simulink model "CSWI"  (Simulink 7.8)
settings: Solver=ode3  StartTime=0.0  StopTime=t_sim  FixedStep=1/6400  MaxStep=0.001  MinStep=0.000005  RelTol=1e-3
StopFcn:
  | ComtradeWrite5( RDRE1_UIabc, RDRE1_ANames, RDRE1_Dsignals, RDRE1_DNames, RDRE1_ADCscale, RDRE1_PromtFile, RDRE1_NumFile, RDRE1_FileFormat, RDRE1_TestNum);
  | clear RDRE1_UIabc RDRE1_ANames RDRE1_Dsignals RDRE1_DNames RDRE1_ADCscale  RDRE1_PromtFile RDRE1_NumFile RDRE1_FileFormat RDRE1_TestNum
values from neighbouring files (symbols this model uses):
  BlkTmms1 = 700    [CSWI_SG1.m]    (also in CSWI_SG2.m = 650; CSWI_SG3.m; CSWI_SG4.m; CSWI_SG5.m)
  BlkTmms2 = 800    [CSWI_SG1.m]    (also in CSWI_SG2.m = 750; CSWI_SG3.m; CSWI_SG4.m; CSWI_SG5.m)
  ClsTmms1 = 250    [CSWI_SG1.m]    (also in CSWI_SG2.m = 200; CSWI_SG3.m; CSWI_SG4.m; CSWI_SG5.m)
  ClsTmms2 = 170    [CSWI_SG1.m]    (also in CSWI_SG2.m = 100; CSWI_SG3.m; CSWI_SG4.m; CSWI_SG5.m)
  ClsTmms3 = 60    [CSWI_SG1.m]    (also in CSWI_SG2.m = 30; CSWI_SG3.m; CSWI_SG4.m; CSWI_SG5.m)
  ClsTmms4 = 10    [CSWI_SG1.m]    (also in CSWI_SG2.m = 20; CSWI_SG3.m; CSWI_SG4.m; CSWI_SG5.m)
  FailTmms = 350    [CSWI_SG1.m]    (also in CSWI_SG2.m = 300; CSWI_SG3.m; CSWI_SG4.m; CSWI_SG5.m)
  FctMod1 = 1    [CSWI_SG1.m]    (also in CSWI_SG2.m; CSWI_SG3.m; CSWI_SG4.m; CSWI_SG5.m)
  FctMod2 = 1    [CSWI_SG1.m]    (also in CSWI_SG2.m; CSWI_SG3.m; CSWI_SG4.m = 0; CSWI_SG5.m)
  FctMod3 = 1    [CSWI_SG1.m]    (also in CSWI_SG2.m; CSWI_SG3.m; CSWI_SG4.m; CSWI_SG5.m = 0)
  Num_SG = 1    [CSWI_generate_tests.m]
  OpnTmms1 = 300    [CSWI_SG1.m]    (also in CSWI_SG2.m = 250; CSWI_SG3.m; CSWI_SG4.m; CSWI_SG5.m)
  OpnTmms2 = 200    [CSWI_SG1.m]    (also in CSWI_SG2.m = 150; CSWI_SG3.m; CSWI_SG4.m; CSWI_SG5.m)
  OpnTmms3 = 30    [CSWI_SG1.m]    (also in CSWI_SG2.m = 90; CSWI_SG3.m = 90; CSWI_SG4.m; CSWI_SG5.m)
  test_dc = 'Ïðîâåðêà îòñóòñòâèÿ ôîðìèðîâàíèÿ ñèãíàëîâ "Âêë." ïðè ôîðìèðîâàíèè ñèãíàëà  "Îòêë. îò ÄÓ"'    [CSWI_generate_tests.m]
undefined symbols (not defined in the file or in its folder): sigbuilder_block, Test_num
libraries: powerlib_extras x21
(part 1 of 3)
settings Model: Creator=ivanovsn  LastModifiedBy=nikonenok

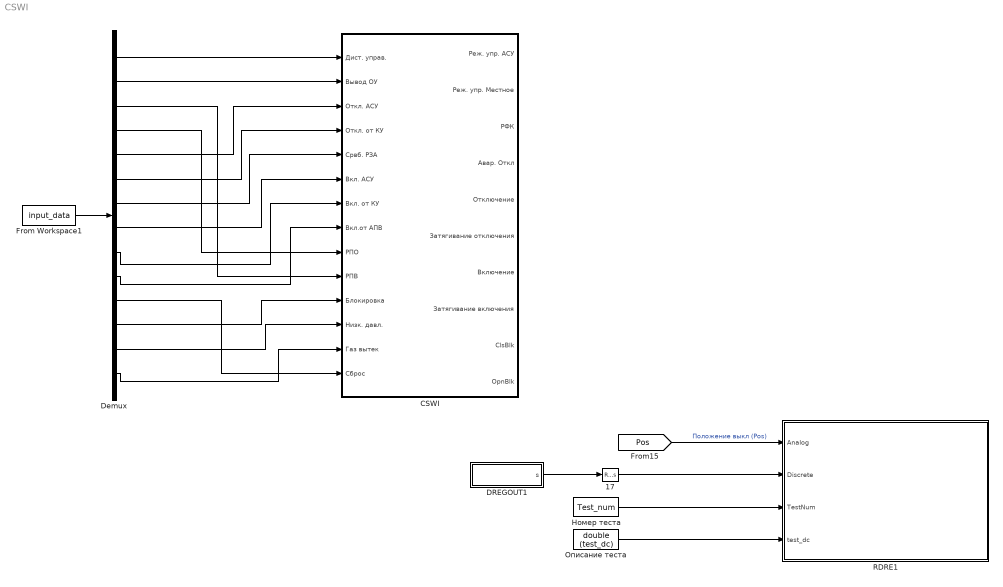
== system CSWI ==
  " 17" : RateTransition  OutPortSampleTime=1/6400
  CSWI : Subsystem  mask(CSWI){OpnTmms1=OpnTmms1, OpnTmms2=OpnTmms2, OpnTmms3=OpnTmms3, ClsTmms1=ClsTmms1, ClsTmms2=ClsTmms2, ClsTmms3=ClsTmms3, ClsTmms4=ClsTmms4, FailTmms=FailTmms, BlkTmms1=BlkTmms1, BlkTmms2=BlkTmms2, FctMod1=FctMod1, FctMod2=FctMod2, FctMod3=FctMod3, Tmega=1/6400}
      mask prompts: OpnTmms1 "Выдержка времени контроля затягивания отключения, мс"; OpnTmms2 "Минимальная длительность сигнала отключения, мс"; OpnTmms3 "Выдержка времени на подхват сигнала отключения, мс"; ClsTmms1 "Выдержка времени контроля затягивания включения, мс"; ClsTmms2 "Минимальная длительность сигнала включения, мс"; ClsTmms3 "Выдержка времени подхвата включения, мс"; ClsTmms4 "Время блокировки команды включения, мс"; FailTmms "Выдержка времени на формирование сигнала аварийного отключения, мс"; BlkTmms1 "Выдержка времени на блокировку формирование команды на включение выключателя при наличии сигнала «Низкое давление элегаза»"; BlkTmms2 "Выдержка времени на блокировку формирование команд на включение и отключение выключателя при наличии сигнала «Элегаз вытек»"; FctMod1 "Ввод режима дистанционного управления при наличии сигнала на входе «InRemCtl»"; FctMod2 "Ввод блокировки команды отключения выключателя при наличии сигнала затягивания отключения"; FctMod3 "Ввод блокировки команды включения выключателя при наличии сигнала затягивания включения"; Tmega "Cycle Time, c"
      mask init:
      | OpnTmms1=OpnTmms1/1000;
      | OpnTmms2=OpnTmms2/1000;
      | OpnTmms3=OpnTmms3/1000;
      | ClsTmms1=ClsTmms1/1000;
      | ClsTmms2=ClsTmms2/1000;
      | ClsTmms3=ClsTmms3/1000;
      | ClsTmms4=ClsTmms4/1000;
      | FailTmms=FailTmms/1000;
      | BlkTmms1=BlkTmms1/1000;
      | BlkTmms2=BlkTmms2/1000;
  DREGOUT1 : Subsystem
  Demux : Demux  Outputs=14
  From Workspace1 : FromWorkspace  VariableName=input_data  OutputAfterFinalValue=Setting to zero
  RDRE1 : Subsystem  mask(RDRE){SamplTime=1/6400, ADCscale=16, FileName=CSWI_test, FileFormat=ASCII}
      mask prompts: SamplTime "Sample time, s"; ADCscale "ADC scale"; FileName "File name"; FileFormat "File format"
      mask help: Сохранение результатов моделирования в формате COMTRADE 1991 (текстовом или бинарном).
      mask init:
      | RDRE_path = gcb;
      | 
      | RDRE_name = get_param (gcb, 'Name');
      | Td = SamplTime;
      | 
      | porthandles = get(gcbh, 'PortHandles');
      | linehandle1 = get(porthandles.Inport(1), 'Line');
      | 
      | if linehandle1 ~= -1
      | set(linehandle1, 'SignalPropagation', 'on');
      | ANames1 = get (porthandles.Inport(1), 'Label');
      | 
      | else ANames1 = 'empty';
      | end
      | 
      | linehandle2 = get(porthandles.Inport(2), 'Line');
      | if linehandle2 ~= -1
      | set(linehandle2, 'SignalPropagation', 'on');
      | DNames1 = get (porthandles.Inport(2), 'Label');
      | 
      | else DNames1 = 'empty';
      | end
      | 
      | 
      | set_param( strcat(RDRE_path, '/' , 'To Workspace'), 'VariableName', 'UIabc' );
      | set_param( strcat(RDRE_path, '/' , 'To Workspace'), 'VariableName', strcat(RDRE_name, '_', 'UIabc'));
      | 
      | set_param( strcat(RDRE_path, '/' , 'To Workspace9'), 'VariableName', 'ANames' );
      | set_param( strcat(RDRE_path, '/' , 'To Workspace9'), 'VariableName', strcat(RDRE_name, '_', 'ANames'));
      | ANames = double (ANames1);
      | 
      | set_param( strcat(RDRE_path, '/' , 'To Workspace1'), 'VariableName', 'ADCscale' );
      | set_param( strcat(RDRE_path, '/' , 'To Workspace1'), 'VariableName', strcat(RDRE_name, '_', 'ADCscale'));
      | 
      | set_param( strcat(RDRE_path, '/' , 'To Workspace11'), 'VariableName', 'PromtFile' );
      | set_param( strcat(RDRE_path, '/' , 'To Workspace11'), 'VariableName', strcat(RDRE_name, '_', 'PromtFile'));
      | % NumPromt = double( PromtFile );
      | 
      | 
      | 
      | set_param( strcat(RDRE_path, '/' , 'To Workspace2'), 'VariableName', 'NumFile' );
      | set_param( strcat(RDRE_path, '/' , 'To Workspace2'), 'VariableName', strcat(RDRE_name, '_', 'NumFile'));
      | NumFile = double( FileName );
      | 
      | set_param( strcat(RDRE_path, '/' , 'To Workspace3'), 'VariableName', 'FileFormat' );
      | set_param( strcat(RDRE_path, '/' , 'To Workspace3'), 'VariableName', strcat(RDRE_name, '_', 'FileFormat'));
      | %FileFormat = double( file_format );
      | 
      | set_param( strcat(RDRE_path, '/' , 'To Workspace4'), 'VariableName', 'Dsignals' );
      | set_param( strcat(RDRE_path, '/' , 'To Workspace4'), 'VariableName', strcat(RDRE_name, '_', 'Dsignals'));
      | 
      | set_param( strcat(RDRE_path, '/' , 'To Workspace10'), 'VariableName', 'DNames' );
      | set_param( strcat(RDRE_path, '/' , 'To Workspace10'), 'VariableName', strcat(RDRE_name, '_', 'DNames'));
      | DNames = double (DNames1);
      | 
      | 
      | Td = SamplTime;
      | 
      | % sys = get_param(bdroot, 'Handle');
      | % l = find_system(sys, 'FindAll', 'on', 'type', 'line')
      | % for i=1:length(l)
      | %       %set(l(i),'signalPropagation','off');
      | %       set(l(i),'signalPropagation','on')
      | % end
      mask Help:
      | Comtrade generator - блок сохранения результатов моделирования в формате COMTRADE
      | (текстовом или бинарном).
      | На входы блока (Analog и Discrete) подаются аналоговые и дискретные сигналы соответственно,
      | объединенные с помощью блоков Mux или Bus Creator.
      | В параметрах блока задаются:
      |  - интервал дискретизации (Sample time);
      |  - разрядность АЦП (ADC scale);
      |  - имя файла осциллограммы (File name);
      |  - заголовок осциллограммы (Promt file);
      |  - формат осциллограммы (File format);
      |  - время записываемого предаварийного режима (Prefault time);
      |  - время записываемого послеаварийного режима (Postfault time);
      |  - длительность записываемой осциллограмы (Limit time);
      |  - Выбор режима записи (Manual). Для выбора РУЧНОГО режима записи
      | необходимо выставить флажок на вкладке MANUAL MODE.
      | В РУЧНОМ режиме осцилограмма записывается с начала (Start time = 0)
      | и ограничивается пользовательским временем симуляции (Stop time)
      | В АВТОМАТИЧЕСКОМ режиме (снять флажок с вкладки MANUAL MODE) осциллограмма ограничивается временами
      | Prefault time, Postfault time, Limit time
      mask StyleString: edit,edit,edit,popup(ASCII|BINARY)
      mask Display: disp( 'WRITE \nCOMTRADE\n\nSNames from labels' )
  Номер теста : Constant  Value=Test_num
  Описание теста : Constant  Value=double (test_dc)
  wires:
  Номер теста/1 -> RDRE1/3(TestNum)
  Описание теста/1 -> RDRE1/4(test_dc)
  DREGOUT1/1(s) -> " 17"/1
  From Workspace1/1 -> Demux/1
  " 17"/1 -> RDRE1/2(Discrete)
  Demux/1 -> CSWI/1(Дист. управ.)
  Demux/2 -> CSWI/2(Вывод ОУ)
  Demux/3 -> CSWI/10(РПВ)
  Demux/4 -> CSWI/9(РПО)
  Demux/5 -> CSWI/3(Откл. АСУ)
  Demux/6 -> CSWI/4(Откл. от КУ)
  Demux/7 -> CSWI/5(Срвб. РЗА)
  Demux/8 -> CSWI/6(Вкл. АСУ)
  Demux/9 -> CSWI/7(Вкл. от КУ)
  Demux/10 -> CSWI/8(Вкл.от АПВ)
  Demux/11 -> CSWI/14(Сброс)
  Demux/12 -> CSWI/11(Блокировка)
  Demux/13 -> CSWI/12(Низк. давл.)
  Demux/14 -> CSWI/13(Газ вытек)
  [Pos] -> RDRE1/1(Analog)  "Положение выкл (Pos)"

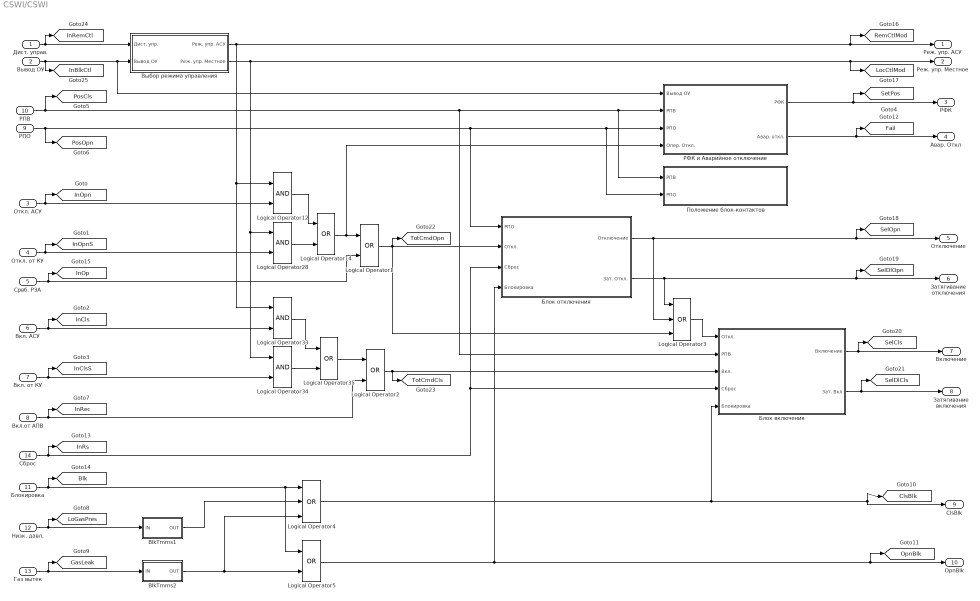
== system CSWI/CSWI ==
  Дист. управ. : Inport  SampleTime=Tmega
  Вывод ОУ : Inport  Port=2  SampleTime=Tmega
  Откл. АСУ : Inport  Port=3  SampleTime=Tmega
  Откл. от КУ : Inport  Port=4  SampleTime=Tmega
  Срвб. РЗА : Inport  Port=5  SampleTime=Tmega
  Вкл. АСУ : Inport  Port=6  SampleTime=Tmega
  Вкл. от КУ : Inport  Port=7  SampleTime=Tmega
  Вкл.от АПВ : Inport  Port=8  SampleTime=Tmega
  РПО : Inport  Port=9  SampleTime=Tmega
  РПВ : Inport  Port=10  SampleTime=Tmega
  Блокировка : Inport  Port=11  SampleTime=Tmega
  Низк. давл. : Inport  Port=12  SampleTime=Tmega
  Газ вытек : Inport  Port=13  SampleTime=Tmega
  Сброс : Inport  Port=14  SampleTime=Tmega
  BlkTmms1 : Subsystem  DialogController=POWERSYS.PowerSysDialog  mask(Discrete On/Off Delay ){type_delay=On delay, delay=BlkTmms1, ic=0, Ts=Tmega}
      mask prompts: type_delay "Type:"; delay "Time delay:"; ic "Input at t = -Ts (0/1):"; Ts "Sample time Ts:"
      mask help:
      | Apply a delay on the input signal when the input changes to TRUE (1) or FALSE (0).
      |
      | On delay: When the input becomes TRUE, the output becomes TRUE after the specified time delay as long as the input is still TRUE. If the input becomes FALSE before the time delay has expired , the output stays FALSE.
      |
      | Off delay: When the input becomes FALSE, the output becomes FALSE after the specified time delay as long as the input is still FALSE. If the input becomes TRUE before the time delay has expired , the output stays TRUE.
      |
      | The input value (0/1) at time step preceding t=0 is specified by the parameter "input at t = -Ts".
      mask init:
      | str=sprintf('%g %c',delay,'s');
      | power_initmask();
      mask Help: This block is part of a subset of blocks in the Extras library that does not have documentation associated with it, other than the block mask description.
      mask StyleString: popup(On delay|Off delay),edit,edit,edit
      mask Display:
      | plot(0,0,100,100,[10,10,10,90,90,90],[60,40,50,50,40,60]);
      | text(25+(type_delay-1)*50,80,'t');
      | text(15,20,str);
  BlkTmms2 : Subsystem  DialogController=POWERSYS.PowerSysDialog  mask(Discrete On/Off Delay ){type_delay=On delay, delay=BlkTmms2, ic=0, Ts=Tmega}
      mask prompts: type_delay "Type:"; delay "Time delay:"; ic "Input at t = -Ts (0/1):"; Ts "Sample time Ts:"
      mask help:
      | Apply a delay on the input signal when the input changes to TRUE (1) or FALSE (0).
      |
      | On delay: When the input becomes TRUE, the output becomes TRUE after the specified time delay as long as the input is still TRUE. If the input becomes FALSE before the time delay has expired , the output stays FALSE.
      |
      | Off delay: When the input becomes FALSE, the output becomes FALSE after the specified time delay as long as the input is still FALSE. If the input becomes TRUE before the time delay has expired , the output stays TRUE.
      |
      | The input value (0/1) at time step preceding t=0 is specified by the parameter "input at t = -Ts".
      mask init:
      | str=sprintf('%g %c',delay,'s');
      | power_initmask();
      mask Help: This block is part of a subset of blocks in the Extras library that does not have documentation associated with it, other than the block mask description.
      mask StyleString: popup(On delay|Off delay),edit,edit,edit
      mask Display:
      | plot(0,0,100,100,[10,10,10,90,90,90],[60,40,50,50,40,60]);
      | text(25+(type_delay-1)*50,80,'t');
      | text(15,20,str);
  Logical Operator{1..2,5,14,35} (5 alike) : Logic  Operator=OR  AllPortsSameDT=off  OutDataTypeStr=boolean  SampleTime=Tmega
  Logical Operator{12,28,33..34} (4 alike) : Logic  AllPortsSameDT=off  OutDataTypeStr=boolean  SampleTime=Tmega
  Logical Operator3 : Logic  Operator=OR  Inputs=3  AllPortsSameDT=off  OutDataTypeStr=boolean  SampleTime=Tmega
  Logical Operator4 : Logic  Operator=OR  Inputs=3  AllPortsSameDT=off  OutDataTypeStr=boolean  SampleTime=Tmega
  Блок включения : Subsystem
  Блок отключения : Subsystem
  Выбор режима управления : Subsystem
  Положение блок-контактов : Subsystem
  РФК и Аварийное отключение : Subsystem
  Реж. упр. АСУ : Outport  SampleTime=Tmega
  Реж. упр. Местное : Outport  Port=2  SampleTime=Tmega
  РФК : Outport  Port=3  SampleTime=Tmega
  Авар. Откл : Outport  Port=4  SampleTime=Tmega
  Отключение : Outport  Port=5  SampleTime=Tmega
  Затягивание отключения : Outport  Port=6  SampleTime=Tmega
  Включение : Outport  Port=7  SampleTime=Tmega
  Затягивание включения : Outport  Port=8  SampleTime=Tmega
  ClsBlk : Outport  Port=9  SampleTime=Tmega
  OpnBlk : Outport  Port=10  SampleTime=Tmega
  tag scope: Blk=global, ClsBlk=global, Fail=global, GasLeak=global, InBlkCtl=global, InCls=global, InClsS=global, InOp=global, InOpn=global, InOpnS=global, InRec=global, InRemCtl=global, InRs=global, LoGasPres=global, LocCtlMod=global, OpnBlk=global, PosCls=global, PosOpn=global, RemCtlMod=global, SelCls=global, SelDlCls=global, SelDlOpn=global, SelOpn=global, SetPos=global, TotCmdCls=global, TotCmdOpn=global
  wires:
  Откл. АСУ/1 -> [InOpn], Logical Operator12/2
  Дист. управ./1 -> Выбор режима управления/1(Дист. упр.), [InRemCtl]
  Откл. от КУ/1 -> [InOpnS], Logical Operator28/2
  Вкл. АСУ/1 -> [InCls], Logical Operator33/2
  Вкл. от КУ/1 -> [InClsS], Logical Operator34/2
  Вывод ОУ/1 -> РФК и Аварийное отключение/1(Вывод ОУ), Выбор режима управления/2(Вывод ОУ), [InBlkCtl]
  РФК и Аварийное отключение/2(Авар. откл.) -> Авар. Откл/1, [Fail]
  РФК и Аварийное отключение/1(РФК) -> РФК/1, [SetPos]
  Выбор режима управления/2(Реж. упр. Местное) -> Logical Operator28/1, Logical Operator34/1, Реж. упр. Местное/1, [LocCtlMod]
  Выбор режима управления/1(Реж. упр. АСУ) -> Logical Operator12/1, Logical Operator33/1, Реж. упр. АСУ/1, [RemCtlMod]
  Logical Operator33/1 -> Logical Operator35/1
  Logical Operator34/1 -> Logical Operator35/2
  Logical Operator28/1 -> Logical Operator14/2
  Logical Operator12/1 -> Logical Operator14/1
  РПВ/1 -> Блок включения/2(РПВ), РФК и Аварийное отключение/2(РПВ), Положение блок-контактов/1(РПВ), [PosCls]
  РПО/1 -> [PosOpn], Блок отключения/1(РПО), РФК и Аварийное отключение/3(РПО), Положение блок-контактов/2(РПО)
  Logical Operator14/1 -> РФК и Аварийное отключение/4(Опер. Откл.), Logical Operator1/1
  Срвб. РЗА/1 -> Logical Operator1/2, [InOp]
  Logical Operator35/1 -> Logical Operator2/1
  Вкл.от АПВ/1 -> [InRec], Logical Operator2/2
  Низк. давл./1 -> [LoGasPres], BlkTmms1/1(IN)
  Газ вытек/1 -> [GasLeak], BlkTmms2/1(IN)
  BlkTmms1/1(OUT) -> Logical Operator4/2
  BlkTmms2/1(OUT) -> Logical Operator5/2, Logical Operator4/3
  Блокировка/1 -> Logical Operator4/1, Logical Operator5/1, [Blk]
  Logical Operator4/1 -> ClsBlk/1, [ClsBlk], Блок включения/5(Блокировка)
  Logical Operator5/1 -> OpnBlk/1, [OpnBlk], Блок отключения/4(Блокировка)
  Logical Operator1/1 -> Блок отключения/2(Откл.), [TotCmdOpn], Logical Operator3/3
  Сброс/1 -> [InRs], Блок отключения/3(Сброс), Блок включения/4(Сброс)
  Logical Operator2/1 -> Блок включения/3(Вкл.), [TotCmdCls]
  Блок включения/1(Включение) -> Включение/1, [SelCls]
  Блок включения/2(Зат. Вкл) -> Затягивание включения/1, [SelDlCls]
  Блок отключения/1(Отключение) -> Отключение/1, [SelOpn], Logical Operator3/2
  Блок отключения/2(Зат. Откл.) -> Затягивание отключения/1, [SelDlOpn], Logical Operator3/1
  Logical Operator3/1 -> Блок включения/1(Откл.)

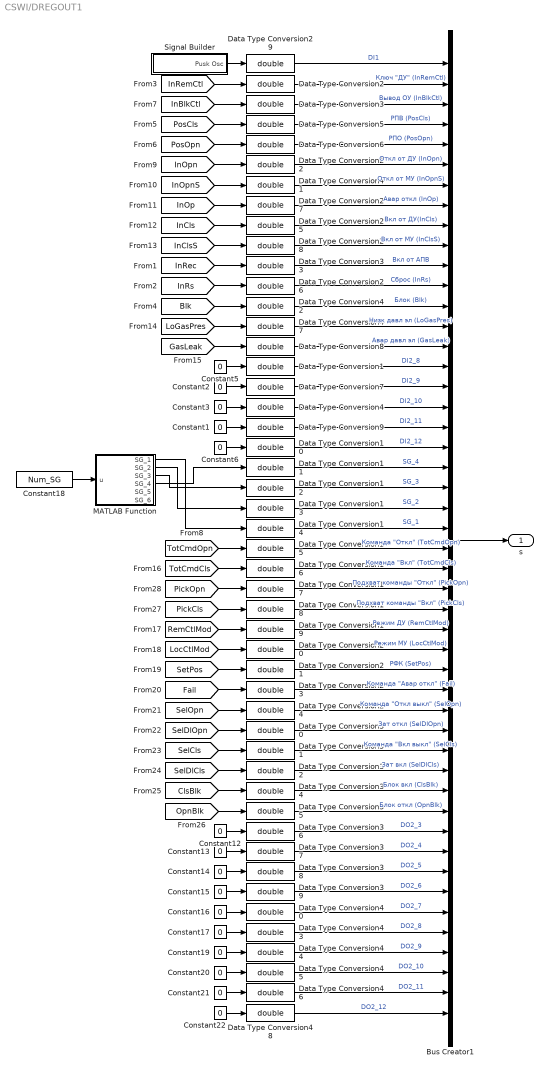
== system CSWI/DREGOUT1 ==
  Bus Creator1 : BusCreator  Inputs=48
  Constant{1..3,5..6,12..17,19..22} (15 alike) : Constant  Value=0
  Constant18 : Constant  Value=Num_SG
  Data Type Conversion{1..48} (48 alike) : DataTypeConversion  OutDataTypeStr=double
  MATLAB Function : MATLAB Function  TreatAsAtomicUnit=on
      settings: RTWSystemCode=Function  RTWFcnNameOpts=Use subsystem name  RTWFileNameOpts=Use subsystem name
  Signal Builder : Subsystem  Tag=STV Subsys  LoadFcn=sigbuilder_block('load');  StartFcn=sigbuilder_block('start');  StopFcn=sigbuilder_block('stop');  ClipboardFcn=sigbuilder_block('clipboard');  mask(Sigbuilder block){}
      mask help: Simulink:masks:SigbuilderBlock_MD
      mask init:
      | if ~strcmp(get_param(bdroot(gcbh),'SimulationStatus'),'stopped') tuvar = sigbuilder_block('maskInit'); end
      settings: CopyFcn=sigbuilder_block('copy');  DeleteFcn=sigbuilder_block('delete');  ModelCloseFcn=sigbuilder_block('modelClose');  PreSaveFcn=sigbuilder_block('preSave');  NameChangeFcn=sigbuilder_block('namechange');  OpenFcn=sigbuilder_block('open',[437.25 199.5 550.5 399.75 ]);  CloseFcn=sigbuilder_block('close');
      mask Display: plot(0, 0, 100, 100,[2, 2, 32, 32, 2], [68, 8, 8, 68, 68],[32, 2], [38, 38], [32, 19, 2],[53, 60, 44], [32, 17, 17, 2],[16, 16, 31, 31]);txt = getActiveGroup(gcbh);text(2, 100, txt,'verticalAlignment', 'top');
  s : Outport
  wires:
  [Blk] -> Data Type Conversion42/1
  [InRs] -> Data Type Conversion26/1
  [LoGasPres] -> Data Type Conversion47/1
  [InOpnS] -> Data Type Conversion41/1
  [InOpn] -> Data Type Conversion22/1
  [PosOpn] -> Data Type Conversion6/1
  [PosCls] -> Data Type Conversion5/1
  [InBlkCtl] -> Data Type Conversion3/1
  [InRemCtl] -> Data Type Conversion2/1
  Constant18/1 -> MATLAB Function/1(u)
  Signal Builder/1(Pusk Osc) -> Data Type Conversion29/1
  Bus Creator1/1 -> s/1
  Constant2/1 -> Data Type Conversion7/1
  Constant5/1 -> Data Type Conversion1/1
  Data Type Conversion29/1 -> Bus Creator1/1  "DI1"
  Data Type Conversion2/1 -> Bus Creator1/2  "Ключ \"ДУ\" (InRemCtl)"
  [InOp] -> Data Type Conversion27/1
  [InCls] -> Data Type Conversion25/1
  [InClsS] -> Data Type Conversion28/1
  [InRec] -> Data Type Conversion33/1
  [GasLeak] -> Data Type Conversion8/1
  Data Type Conversion6/1 -> Bus Creator1/5  "РПО (PosOpn)"
  Data Type Conversion5/1 -> Bus Creator1/4  "РПВ (PosCls)"
  Data Type Conversion3/1 -> Bus Creator1/3  "Вывод ОУ (InBlkCtl)"
  Data Type Conversion22/1 -> Bus Creator1/6  "Откл от ДУ (InOpn)"
  Data Type Conversion41/1 -> Bus Creator1/7  "Откл от МУ (InOpnS)"
  Data Type Conversion27/1 -> Bus Creator1/8  "Авар откл (InOp)"
  Data Type Conversion25/1 -> Bus Creator1/9  "Вкл от ДУ(InCls)"
  Data Type Conversion28/1 -> Bus Creator1/10  "Вкл от МУ (InClsS)"
  Data Type Conversion33/1 -> Bus Creator1/11  "Вкл от АПВ"
  Data Type Conversion26/1 -> Bus Creator1/12  "Сброс (InRs)"
  Data Type Conversion42/1 -> Bus Creator1/13  "Блок (Blk)"
  Data Type Conversion47/1 -> Bus Creator1/14  "Низк давл эл (LoGasPres)"
  Data Type Conversion8/1 -> Bus Creator1/15  "Авар давл эл (GasLeak)"
  Data Type Conversion1/1 -> Bus Creator1/16  "DI2_8"
  Data Type Conversion7/1 -> Bus Creator1/17  "DI2_9"
  Constant1/1 -> Data Type Conversion9/1
  MATLAB Function/4(SG_4) -> Data Type Conversion11/1
  MATLAB Function/2(SG_2) -> Data Type Conversion13/1
  Constant6/1 -> Data Type Conversion10/1
  Constant3/1 -> Data Type Conversion4/1
  MATLAB Function/3(SG_3) -> Data Type Conversion12/1
  MATLAB Function/1(SG_1) -> Data Type Conversion14/1
  Data Type Conversion4/1 -> Bus Creator1/18  "DI2_10"
  Data Type Conversion9/1 -> Bus Creator1/19  "DI2_11"
  Data Type Conversion10/1 -> Bus Creator1/20  "DI2_12"
  Data Type Conversion11/1 -> Bus Creator1/21  "SG_4"
  Data Type Conversion12/1 -> Bus Creator1/22  "SG_3"
  Data Type Conversion13/1 -> Bus Creator1/23  "SG_2"
  Data Type Conversion14/1 -> Bus Creator1/24  "SG_1"
  Data Type Conversion15/1 -> Bus Creator1/25  "Команда \"Откл\" (TotCmdOpn)"
  [TotCmdOpn] -> Data Type Conversion15/1
  [TotCmdCls] -> Data Type Conversion16/1
  Data Type Conversion16/1 -> Bus Creator1/26  "Команда \"Вкл\" (TotCmdCls)"
  [ClsBlk] -> Data Type Conversion34/1
  [OpnBlk] -> Data Type Conversion35/1
  Constant12/1 -> Data Type Conversion36/1
  Constant13/1 -> Data Type Conversion37/1
  Constant14/1 -> Data Type Conversion38/1
  Constant15/1 -> Data Type Conversion39/1
  Data Type Conversion17/1 -> Bus Creator1/27  "Подхват команды \"Откл\" (PickOpn)"
  Data Type Conversion18/1 -> Bus Creator1/28  "Подхват команды \"Вкл\" (PickCls)"
  Data Type Conversion19/1 -> Bus Creator1/29  "Режим ДУ (RemCtlMod)"
  Data Type Conversion20/1 -> Bus Creator1/30  "Режим МУ (LocCtlMod)"
  Data Type Conversion21/1 -> Bus Creator1/31  "РФК (SetPos)"
  Data Type Conversion23/1 -> Bus Creator1/32  "Команда \"Авар откл\" (Fail)"
  Data Type Conversion24/1 -> Bus Creator1/33  "Команда \"Откл выкл\" (SelOpn)"
  Data Type Conversion30/1 -> Bus Creator1/34  "Зат откл (SelDlOpn)"
  Data Type Conversion31/1 -> Bus Creator1/35  "Команда \"Вкл выкл\" (SelCls)"
  Data Type Conversion32/1 -> Bus Creator1/36  "Зат вкл (SelDlCls)"
  Data Type Conversion34/1 -> Bus Creator1/37  "Блок вкл (ClsBlk)"
  Data Type Conversion35/1 -> Bus Creator1/38  "Блок откл (OpnBlk)"
  Data Type Conversion36/1 -> Bus Creator1/39  "DO2_3"
  Data Type Conversion37/1 -> Bus Creator1/40  "DO2_4"
  Data Type Conversion38/1 -> Bus Creator1/41  "DO2_5"
  Data Type Conversion39/1 -> Bus Creator1/42  "DO2_6"
  Data Type Conversion40/1 -> Bus Creator1/43  "DO2_7"
  Data Type Conversion43/1 -> Bus Creator1/44  "DO2_8"
  Data Type Conversion44/1 -> Bus Creator1/45  "DO2_9"
  Data Type Conversion45/1 -> Bus Creator1/46  "DO2_10"
  Data Type Conversion46/1 -> Bus Creator1/47  "DO2_11"
  Data Type Conversion48/1 -> Bus Creator1/48  "DO2_12"
  Constant16/1 -> Data Type Conversion40/1
  Constant17/1 -> Data Type Conversion43/1
  Constant19/1 -> Data Type Conversion44/1
  Constant20/1 -> Data Type Conversion45/1
  Constant21/1 -> Data Type Conversion46/1
  Constant22/1 -> Data Type Conversion48/1
  [PickOpn] -> Data Type Conversion17/1
  [PickCls] -> Data Type Conversion18/1
  [RemCtlMod] -> Data Type Conversion19/1
  [LocCtlMod] -> Data Type Conversion20/1
  [SetPos] -> Data Type Conversion21/1
  [Fail] -> Data Type Conversion23/1
  [SelOpn] -> Data Type Conversion24/1
  [SelDlOpn] -> Data Type Conversion30/1
  [SelCls] -> Data Type Conversion31/1
  [SelDlCls] -> Data Type Conversion32/1

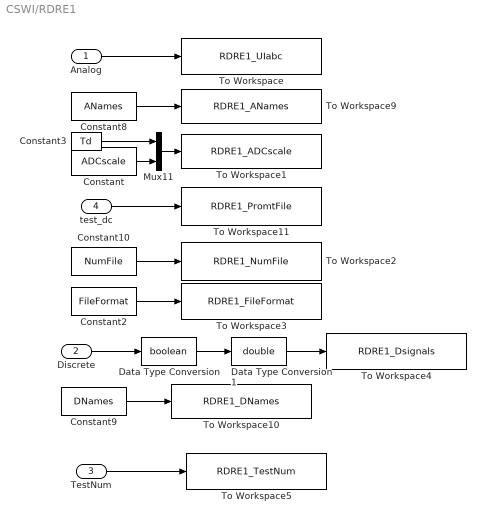
== system CSWI/RDRE1 ==
  Analog : Inport
  Discrete : Inport  Port=2
  TestNum : Inport  Port=3
  test_dc : Inport  Port=4
  Constant : Constant  Value=ADCscale
  Constant10 : Constant  Value=NumFile
  Constant2 : Constant  Value=FileFormat
  Constant3 : Constant  Value=Td
  Constant8 : Constant  Value=ANames
  Constant9 : Constant  Value=DNames
  Data Type Conversion : DataTypeConversion  OutDataTypeStr=boolean  RndMeth=Zero
  Data Type Conversion1 : DataTypeConversion  OutDataTypeStr=double  RndMeth=Zero
  Mux11 : Mux  Inputs=2
  To Workspace : ToWorkspace  VariableName=RDRE1_UIabc  SampleTime=Td  SaveFormat=Structure With Time
  To Workspace1 : ToWorkspace  VariableName=RDRE1_ADCscale  SampleTime=1.e3  SaveFormat=Array
  To Workspace10 : ToWorkspace  VariableName=RDRE1_DNames  SampleTime=1.e3  SaveFormat=Array
  To Workspace11 : ToWorkspace  VariableName=RDRE1_PromtFile  SampleTime=1.e3  SaveFormat=Array
  To Workspace2 : ToWorkspace  VariableName=RDRE1_NumFile  SampleTime=1.e3  SaveFormat=Array
  To Workspace3 : ToWorkspace  VariableName=RDRE1_FileFormat  SampleTime=1.e3  SaveFormat=Array
  To Workspace4 : ToWorkspace  VariableName=RDRE1_Dsignals  SampleTime=Td  SaveFormat=Structure With Time
  To Workspace5 : ToWorkspace  VariableName=RDRE1_TestNum  SampleTime=Td  SaveFormat=Array
  To Workspace9 : ToWorkspace  VariableName=RDRE1_ANames  SampleTime=1.e3  SaveFormat=Array
  wires:
  test_dc/1 -> To Workspace11/1
  Constant10/1 -> To Workspace2/1
  Constant8/1 -> To Workspace9/1
  Constant9/1 -> To Workspace10/1
  Constant2/1 -> To Workspace3/1
  Constant3/1 -> Mux11/1
  Mux11/1 -> To Workspace1/1
  Constant/1 -> Mux11/2
  Discrete/1 -> Data Type Conversion/1
  Data Type Conversion/1 -> Data Type Conversion1/1
  Data Type Conversion1/1 -> To Workspace4/1
  Analog/1 -> To Workspace/1
  TestNum/1 -> To Workspace5/1

== system CSWI/CSWI/BlkTmms1 ==
  note: Silvano Casoria
      | Power System Simulation Laboratory
      | IREQ, Hydro-Quebc
  note: Discrete On/Off Delay
  IN : Inport  SampleTime=Tmega
  Constant : Constant  SampleTime=Tmega
  Constant1 : Constant  Value=delay - eps  SampleTime=Tmega
  Constant2 : Constant  Value=type_delay  SampleTime=Tmega
  Data Type Conversion1 : DataTypeConversion  OutDataTypeStr=boolean  SampleTime=Tmega  SaturateOnIntegerOverflow=on  RndMeth=Zero
  Logical Operator1 : Logic  Operator=OR  SampleTime=Tmega
  Logical Operator2 : Logic  Operator=NOT  Inputs=1  SampleTime=Tmega
  OFF Delay : Subsystem  TreatAsAtomicUnit=on
  ON Delay : Subsystem  TreatAsAtomicUnit=on
  Relational Operator1 : RelationalOperator  Operator===  SampleTime=Tmega  InputSameDT=on
  OUT : Outport  SampleTime=Tmega
  wires:
  Data Type Conversion1/1 -> ON Delay/1(IN), OFF Delay/1(IN)
  Constant/1 -> Relational Operator1/2
  Relational Operator1/1 -> ON Delay/Enable, Logical Operator2/1
  Constant2/1 -> Relational Operator1/1
  Logical Operator2/1 -> OFF Delay/Enable
  OFF Delay/1(OUT) -> Logical Operator1/2
  ON Delay/1(OUT) -> Logical Operator1/1
  Logical Operator1/1 -> OUT/1
  Constant1/1 -> ON Delay/2(DELAY), OFF Delay/2(DELAY)
  IN/1 -> Data Type Conversion1/1

== system CSWI/CSWI/BlkTmms2 ==
  note: Silvano Casoria
      | Power System Simulation Laboratory
      | IREQ, Hydro-Quebc
  note: Discrete On/Off Delay
  IN : Inport  SampleTime=Tmega
  Constant : Constant  SampleTime=Tmega
  Constant1 : Constant  Value=delay - eps  SampleTime=Tmega
  Constant2 : Constant  Value=type_delay  SampleTime=Tmega
  Data Type Conversion1 : DataTypeConversion  OutDataTypeStr=boolean  SampleTime=Tmega  SaturateOnIntegerOverflow=on  RndMeth=Zero
  Logical Operator1 : Logic  Operator=OR  SampleTime=Tmega
  Logical Operator2 : Logic  Operator=NOT  Inputs=1  SampleTime=Tmega
  OFF Delay : Subsystem  TreatAsAtomicUnit=on
  ON Delay : Subsystem  TreatAsAtomicUnit=on
  Relational Operator1 : RelationalOperator  Operator===  SampleTime=Tmega  InputSameDT=on
  OUT : Outport  SampleTime=Tmega
  wires:
  Data Type Conversion1/1 -> ON Delay/1(IN), OFF Delay/1(IN)
  Constant/1 -> Relational Operator1/2
  Relational Operator1/1 -> ON Delay/Enable, Logical Operator2/1
  Constant2/1 -> Relational Operator1/1
  Logical Operator2/1 -> OFF Delay/Enable
  OFF Delay/1(OUT) -> Logical Operator1/2
  ON Delay/1(OUT) -> Logical Operator1/1
  Logical Operator1/1 -> OUT/1
  Constant1/1 -> ON Delay/2(DELAY), OFF Delay/2(DELAY)
  IN/1 -> Data Type Conversion1/1

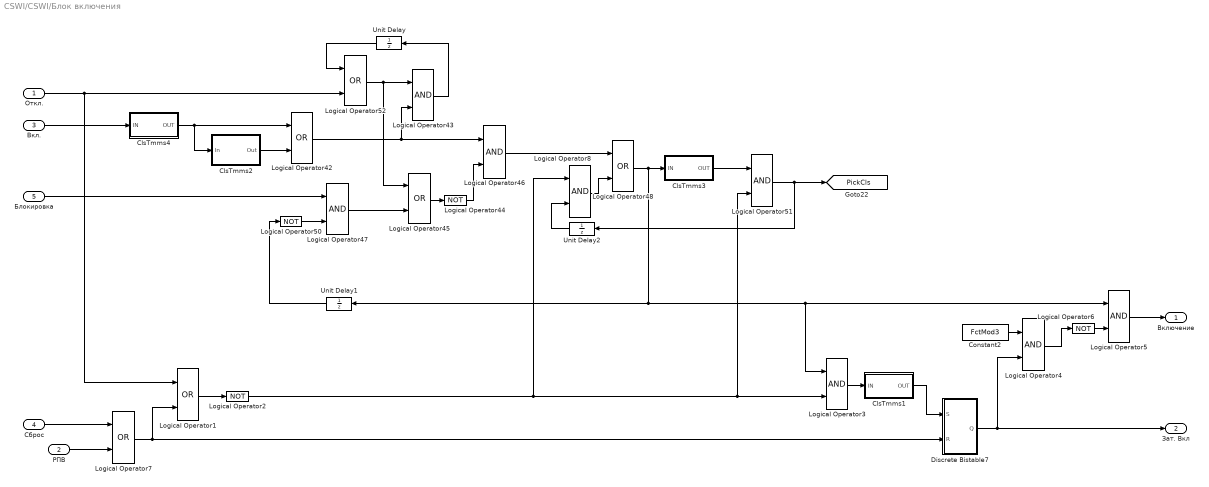
== system CSWI/CSWI/Блок включения ==
  Откл. : Inport  SampleTime=Tmega
  РПВ : Inport  Port=2  SampleTime=Tmega
  Вкл. : Inport  Port=3  SampleTime=Tmega
  Сброс : Inport  Port=4  SampleTime=Tmega
  Блокировка : Inport  Port=5  SampleTime=Tmega
  ClsTmms1 : Subsystem  DialogController=POWERSYS.PowerSysDialog  mask(Discrete On/Off Delay ){type_delay=On delay, delay=ClsTmms1, ic=0, Ts=Tmega}
      mask prompts: type_delay "Type:"; delay "Time delay:"; ic "Input at t = -Ts (0/1):"; Ts "Sample time Ts:"
      mask help:
      | Apply a delay on the input signal when the input changes to TRUE (1) or FALSE (0).
      |
      | On delay: When the input becomes TRUE, the output becomes TRUE after the specified time delay as long as the input is still TRUE. If the input becomes FALSE before the time delay has expired , the output stays FALSE.
      |
      | Off delay: When the input becomes FALSE, the output becomes FALSE after the specified time delay as long as the input is still FALSE. If the input becomes TRUE before the time delay has expired , the output stays TRUE.
      |
      | The input value (0/1) at time step preceding t=0 is specified by the parameter "input at t = -Ts".
      mask init:
      | str=sprintf('%g %c',delay,'s');
      | power_initmask();
      mask Help: This block is part of a subset of blocks in the Extras library that does not have documentation associated with it, other than the block mask description.
      mask StyleString: popup(On delay|Off delay),edit,edit,edit
      mask Display:
      | plot(0,0,100,100,[10,10,10,90,90,90],[60,40,50,50,40,60]);
      | text(25+(type_delay-1)*50,80,'t');
      | text(15,20,str);
  ClsTmms2 : Subsystem  DialogController=POWERSYS.PowerSysDialog  mask(Discrete Monostable Flip-Flop){EdgeDetect=Rising, t_mono=ClsTmms2, ic=0, Ts=Tmega}
      mask prompts: EdgeDetect "Edge detection"; t_mono "Pulse duration (s):"; ic "Input at t = -Ts:"; Ts "Sample time Ts:"
      mask help:
      | After being triggered  by the specified edge (Rising, Falling or Either), this block outputs a pulse (TRUE signal) for the time specified by parameter "Pulse duration".
      | If the specified edge is detected while the output is TRUE, the monostable is not retriggered
      |
      | The input value (0/1) at time step preceding t = 0 is specified by the parameter "input at t = -Ts.
      mask init:
      | str=sprintf('%g %c',t_mono,'s');
      | if (EdgeDetect ~=3)
      |     x1 = (EdgeDetect -1)*10;
      |     x2 = (EdgeDetect -1)*30;
      | 	X1=[15-8,25,25,35+8]+0; Y1=[65+x2,65+x2,95-x2,95-x2];
      | 	X2=[15,25,35]+0;   Y2=[75+x1,85-x1,75+x1];
      | 	X3=[];X4=[];Y3=[];Y4=[];	
      | else
      | 	x1 = 10;
      | 	x2 = 30;
      | 	X1=[15,25,25,35]-14;  Y1=[65,65,95,95];
      | 	X2=[15,25,35]-14;    Y2=[75,85,75];
      | 	X3=[15,25,25,35]+14; Y3=[65+x2,65+x2,95-x2,95-x2];
      | 	X4=[15,25,35]+14;   Y4=[75+x1,85-x1,75+x1];
      | end
      | power_initmask();
      mask Help: This block is part of a subset of blocks in the Extras library that does not have documentation associated with it, other than the block mask description.
      mask StyleString: popup(Rising|Falling|Either),edit,edit,edit
      mask Display:
      | plot(0,0,100,100,[100 75 75 25 25 0],[25 25 50 50 25 25]-0,X1,Y1,X2,Y2,X3,Y3,X4,Y4);
      | text(45,37,'T');
      | text(15,15,str);
  ClsTmms3 : Subsystem  DialogController=POWERSYS.PowerSysDialog  mask(Discrete On/Off Delay ){type_delay=On delay, delay=ClsTmms3, ic=0, Ts=Tmega}
      mask prompts: type_delay "Type:"; delay "Time delay:"; ic "Input at t = -Ts (0/1):"; Ts "Sample time Ts:"
      mask help:
      | Apply a delay on the input signal when the input changes to TRUE (1) or FALSE (0).
      |
      | On delay: When the input becomes TRUE, the output becomes TRUE after the specified time delay as long as the input is still TRUE. If the input becomes FALSE before the time delay has expired , the output stays FALSE.
      |
      | Off delay: When the input becomes FALSE, the output becomes FALSE after the specified time delay as long as the input is still FALSE. If the input becomes TRUE before the time delay has expired , the output stays TRUE.
      |
      | The input value (0/1) at time step preceding t=0 is specified by the parameter "input at t = -Ts".
      mask init:
      | str=sprintf('%g %c',delay,'s');
      | power_initmask();
      mask Help: This block is part of a subset of blocks in the Extras library that does not have documentation associated with it, other than the block mask description.
      mask StyleString: popup(On delay|Off delay),edit,edit,edit
      mask Display:
      | plot(0,0,100,100,[10,10,10,90,90,90],[60,40,50,50,40,60]);
      | text(25+(type_delay-1)*50,80,'t');
      | text(15,20,str);
  ClsTmms4 : Subsystem  DialogController=POWERSYS.PowerSysDialog  mask(Discrete On/Off Delay ){type_delay=On delay, delay=ClsTmms4, ic=0, Ts=Tmega}
      mask prompts: type_delay "Type:"; delay "Time delay:"; ic "Input at t = -Ts (0/1):"; Ts "Sample time Ts:"
      mask help:
      | Apply a delay on the input signal when the input changes to TRUE (1) or FALSE (0).
      |
      | On delay: When the input becomes TRUE, the output becomes TRUE after the specified time delay as long as the input is still TRUE. If the input becomes FALSE before the time delay has expired , the output stays FALSE.
      |
      | Off delay: When the input becomes FALSE, the output becomes FALSE after the specified time delay as long as the input is still FALSE. If the input becomes TRUE before the time delay has expired , the output stays TRUE.
      |
      | The input value (0/1) at time step preceding t=0 is specified by the parameter "input at t = -Ts".
      mask init:
      | str=sprintf('%g %c',delay,'s');
      | power_initmask();
      mask Help: This block is part of a subset of blocks in the Extras library that does not have documentation associated with it, other than the block mask description.
      mask StyleString: popup(On delay|Off delay),edit,edit,edit
      mask Display:
      | plot(0,0,100,100,[10,10,10,90,90,90],[60,40,50,50,40,60]);
      | text(25+(type_delay-1)*50,80,'t');
      | text(15,20,str);
  Constant2 : Constant  Value=FctMod3  SampleTime=Tmega
  Discrete Bistable7 : Subsystem  DialogController=POWERSYS.PowerSysDialog  mask(Discrete Bistable Flip-Flop (Priority to Set or Reset)){SPSpriority=Reset, ic=0, Ts=Tmega}
      mask prompts: SPSpriority "Priority to input:"; ic "Initial Q output (0/1):"; Ts "Sample time:"
      mask help:
      | SR Flip-Flop block, with priority given either  to the Set  (S) or Reset  (R) input.
      |
      | Priority to Set: If inputs S (set) and R (reset) are TRUE (1) simultaneously, the output Q is set to TRUE (1).
      |
      | Priority to Reset: If inputs S (set) and R (reset) are TRUE (1) simultaneously, the output Q is reset to FALSE (0).
      |
      | The  Q! output  is the complement of the Q output.
      | The initial value of the Q output  is specified by the parameter "Initial Q output".
      mask init:
      | if (SPSpriority==1)   % RESET
      |  str1 = '[R]';
      |  str2 = 'S';
      | else
      | str1= 'R';
      | str2 = '[S]';
      | end
      | power_initmask();
      mask Help: This block is part of a subset of blocks in the Extras library that does not have documentation associated with it, other than the block mask description.
      mask StyleString: popup(Reset|Set),edit,edit
      mask Display:
      | plot(0,0,100,100);
      | text(8,25,str1);
      | text(8,75,str2);
      | text(72,50,'Q');
  Logical Operator{1,7,42,45,48,52} (6 alike) : Logic  Operator=OR  AllPortsSameDT=off  OutDataTypeStr=boolean  SampleTime=Tmega
  Logical Operator{2,6,44,50} (4 alike) : Logic  Operator=NOT  AllPortsSameDT=off  OutDataTypeStr=boolean  SampleTime=Tmega
  Logical Operator{3..5,8,43,46..47,51} (8 alike) : Logic  AllPortsSameDT=off  OutDataTypeStr=boolean  SampleTime=Tmega
  Unit Delay : UnitDelay  SampleTime=Tmega
  Unit Delay1 : UnitDelay  SampleTime=Tmega
  Unit Delay2 : UnitDelay  SampleTime=Tmega
  Включение : Outport  SampleTime=Tmega
  Зат. Вкл : Outport  Port=2  SampleTime=Tmega
  tag scope: PickCls=global
  wires:
  Logical Operator50/1 -> Logical Operator47/2
  Logical Operator51/1 -> Unit Delay2/1, [PickCls]
  ClsTmms3/1(OUT) -> Logical Operator51/1
  Unit Delay1/1 -> Logical Operator50/1
  Logical Operator48/1 -> ClsTmms3/1(IN), Unit Delay1/1, Logical Operator3/1, Logical Operator5/1
  Logical Operator47/1 -> Logical Operator45/2
  Logical Operator44/1 -> Logical Operator46/2
  Logical Operator45/1 -> Logical Operator44/1
  Logical Operator43/1 -> Unit Delay/1
  Unit Delay/1 -> Logical Operator52/1
  Logical Operator42/1 -> Logical Operator46/1, Logical Operator43/2
  Logical Operator52/1 -> Logical Operator43/1, Logical Operator45/1
  ClsTmms2/1(Out) -> Logical Operator42/2
  ClsTmms4/1(OUT) -> Logical Operator42/1, ClsTmms2/1(In)
  Откл./1 -> Logical Operator52/2, Logical Operator1/1
  Вкл./1 -> ClsTmms4/1(IN)
  Блокировка/1 -> Logical Operator47/1
  Logical Operator1/1 -> Logical Operator2/1
  РПВ/1 -> Logical Operator7/2
  Сброс/1 -> Logical Operator7/1
  Logical Operator2/1 -> Logical Operator3/2, Logical Operator51/2, Logical Operator8/1
  Logical Operator3/1 -> ClsTmms1/1(IN)
  Constant2/1 -> Logical Operator4/1
  Logical Operator4/1 -> Logical Operator6/1
  Logical Operator6/1 -> Logical Operator5/2
  Logical Operator5/1 -> Включение/1
  Logical Operator7/1 -> Logical Operator1/2, Discrete Bistable7/2(R)
  ClsTmms1/1(OUT) -> Discrete Bistable7/1(S)
  Discrete Bistable7/1(Q) -> Logical Operator4/2, Зат. Вкл/1
  Logical Operator46/1 -> Logical Operator48/1
  Logical Operator8/1 -> Logical Operator48/2
  Unit Delay2/1 -> Logical Operator8/2

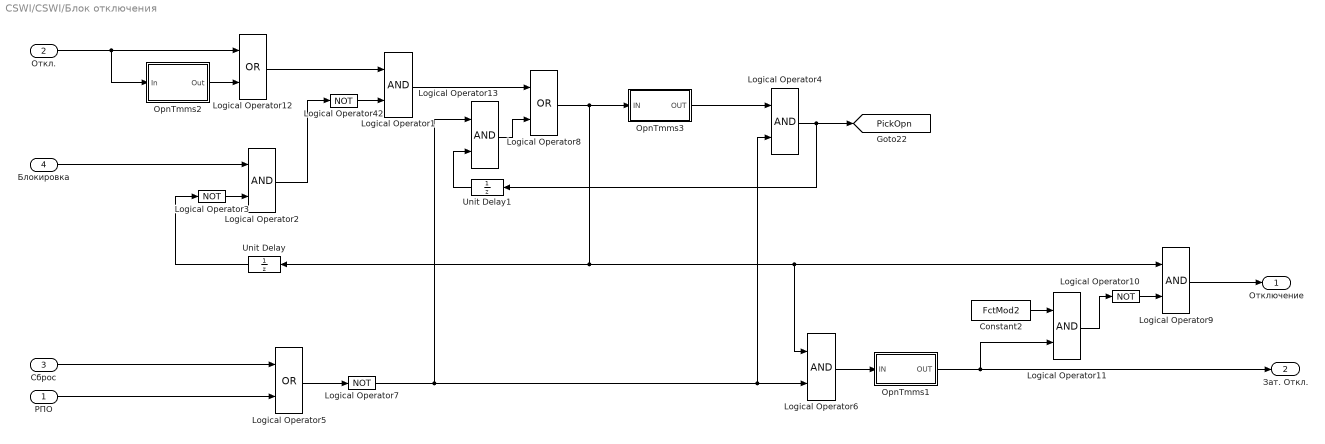
== system CSWI/CSWI/Блок отключения ==
  РПО : Inport  SampleTime=Tmega
  Откл. : Inport  Port=2  SampleTime=Tmega
  Сброс : Inport  Port=3  SampleTime=Tmega
  Блокировка : Inport  Port=4  SampleTime=Tmega
  Constant2 : Constant  Value=FctMod2  SampleTime=Tmega
  Logical Operator{1..2,4,6,9,11,13} (7 alike) : Logic  AllPortsSameDT=off  OutDataTypeStr=boolean  SampleTime=Tmega
  Logical Operator{3,7,10,42} (4 alike) : Logic  Operator=NOT  AllPortsSameDT=off  OutDataTypeStr=boolean  SampleTime=Tmega
  Logical Operator12 : Logic  Operator=OR  AllPortsSameDT=off  OutDataTypeStr=boolean  SampleTime=Tmega
  Logical Operator5 : Logic  Operator=OR  AllPortsSameDT=off  OutDataTypeStr=boolean  SampleTime=Tmega
  Logical Operator8 : Logic  Operator=OR  AllPortsSameDT=off  OutDataTypeStr=boolean  SampleTime=Tmega
  OpnTmms1 : Subsystem  DialogController=POWERSYS.PowerSysDialog  mask(Discrete On/Off Delay ){type_delay=On delay, delay=OpnTmms1, ic=0, Ts=Tmega}
      mask prompts: type_delay "Type:"; delay "Time delay:"; ic "Input at t = -Ts (0/1):"; Ts "Sample time Ts:"
      mask help:
      | Apply a delay on the input signal when the input changes to TRUE (1) or FALSE (0).
      |
      | On delay: When the input becomes TRUE, the output becomes TRUE after the specified time delay as long as the input is still TRUE. If the input becomes FALSE before the time delay has expired , the output stays FALSE.
      |
      | Off delay: When the input becomes FALSE, the output becomes FALSE after the specified time delay as long as the input is still FALSE. If the input becomes TRUE before the time delay has expired , the output stays TRUE.
      |
      | The input value (0/1) at time step preceding t=0 is specified by the parameter "input at t = -Ts".
      mask init:
      | str=sprintf('%g %c',delay,'s');
      | power_initmask();
      mask Help: This block is part of a subset of blocks in the Extras library that does not have documentation associated with it, other than the block mask description.
      mask StyleString: popup(On delay|Off delay),edit,edit,edit
      mask Display:
      | plot(0,0,100,100,[10,10,10,90,90,90],[60,40,50,50,40,60]);
      | text(25+(type_delay-1)*50,80,'t');
      | text(15,20,str);
  OpnTmms2 : Subsystem  DialogController=POWERSYS.PowerSysDialog  mask(Discrete Monostable Flip-Flop){EdgeDetect=Rising, t_mono=OpnTmms2, ic=0, Ts=Tmega}
      mask prompts: EdgeDetect "Edge detection"; t_mono "Pulse duration (s):"; ic "Input at t = -Ts:"; Ts "Sample time Ts:"
      mask help:
      | After being triggered  by the specified edge (Rising, Falling or Either), this block outputs a pulse (TRUE signal) for the time specified by parameter "Pulse duration".
      | If the specified edge is detected while the output is TRUE, the monostable is not retriggered
      |
      | The input value (0/1) at time step preceding t = 0 is specified by the parameter "input at t = -Ts.
      mask init: same as CSWI/CSWI/Блок включения/ClsTmms2
      mask Help: This block is part of a subset of blocks in the Extras library that does not have documentation associated with it, other than the block mask description.
      mask StyleString: popup(Rising|Falling|Either),edit,edit,edit
      mask Display:
      | plot(0,0,100,100,[100 75 75 25 25 0],[25 25 50 50 25 25]-0,X1,Y1,X2,Y2,X3,Y3,X4,Y4);
      | text(45,37,'T');
      | text(15,15,str);
  OpnTmms3 : Subsystem  DialogController=POWERSYS.PowerSysDialog  mask(Discrete On/Off Delay ){type_delay=On delay, delay=OpnTmms3, ic=0, Ts=Tmega}
      mask prompts: type_delay "Type:"; delay "Time delay:"; ic "Input at t = -Ts (0/1):"; Ts "Sample time Ts:"
      mask help:
      | Apply a delay on the input signal when the input changes to TRUE (1) or FALSE (0).
      |
      | On delay: When the input becomes TRUE, the output becomes TRUE after the specified time delay as long as the input is still TRUE. If the input becomes FALSE before the time delay has expired , the output stays FALSE.
      |
      | Off delay: When the input becomes FALSE, the output becomes FALSE after the specified time delay as long as the input is still FALSE. If the input becomes TRUE before the time delay has expired , the output stays TRUE.
      |
      | The input value (0/1) at time step preceding t=0 is specified by the parameter "input at t = -Ts".
      mask init:
      | str=sprintf('%g %c',delay,'s');
      | power_initmask();
      mask Help: This block is part of a subset of blocks in the Extras library that does not have documentation associated with it, other than the block mask description.
      mask StyleString: popup(On delay|Off delay),edit,edit,edit
      mask Display:
      | plot(0,0,100,100,[10,10,10,90,90,90],[60,40,50,50,40,60]);
      | text(25+(type_delay-1)*50,80,'t');
      | text(15,20,str);
  Unit Delay : UnitDelay  SampleTime=Tmega
  Unit Delay1 : UnitDelay  SampleTime=Tmega
  Отключение : Outport  SampleTime=Tmega
  Зат. Откл. : Outport  Port=2  SampleTime=Tmega
  tag scope: PickOpn=global
  wires:
  Logical Operator42/1 -> Logical Operator1/2
  Блокировка/1 -> Logical Operator2/1
  Logical Operator3/1 -> Logical Operator2/2
  Logical Operator2/1 -> Logical Operator42/1
  Unit Delay/1 -> Logical Operator3/1
  Откл./1 -> OpnTmms2/1(In), Logical Operator12/1
  OpnTmms3/1(OUT) -> Logical Operator4/1
  Logical Operator4/1 -> [PickOpn], Unit Delay1/1
  РПО/1 -> Logical Operator5/2
  Logical Operator9/1 -> Отключение/1
  Logical Operator10/1 -> Logical Operator9/2
  Constant2/1 -> Logical Operator11/1
  Logical Operator11/1 -> Logical Operator10/1
  Logical Operator6/1 -> OpnTmms1/1(IN)
  Logical Operator5/1 -> Logical Operator7/1
  Logical Operator7/1 -> Logical Operator13/1, Logical Operator6/2, Logical Operator4/2
  OpnTmms1/1(OUT) -> Logical Operator11/2, Зат. Откл./1
  Logical Operator12/1 -> Logical Operator1/1
  OpnTmms2/1(Out) -> Logical Operator12/2
  Сброс/1 -> Logical Operator5/1
  Logical Operator8/1 -> OpnTmms3/1(IN), Unit Delay/1, Logical Operator9/1, Logical Operator6/1
  Logical Operator1/1 -> Logical Operator8/1
  Logical Operator13/1 -> Logical Operator8/2
  Unit Delay1/1 -> Logical Operator13/2

== system CSWI/CSWI/Выбор режима управления ==
  Дист. упр. : Inport  SampleTime=Tmega
  Вывод ОУ : Inport  Port=2  SampleTime=Tmega
  Constant2 : Constant  Value=FctMod1  SampleTime=Tmega
  Logical Operator27 : Logic  AllPortsSameDT=off  OutDataTypeStr=boolean  SampleTime=Tmega
  Logical Operator32 : Logic  Operator=NOT  AllPortsSameDT=off  OutDataTypeStr=boolean  SampleTime=Tmega
  Logical Operator36 : Logic  AllPortsSameDT=off  OutDataTypeStr=boolean  SampleTime=Tmega
  Logical Operator37 : Logic  AllPortsSameDT=off  OutDataTypeStr=boolean  SampleTime=Tmega
  Logical Operator38 : Logic  Operator=NOT  AllPortsSameDT=off  OutDataTypeStr=boolean  SampleTime=Tmega
  Реж. упр. АСУ : Outport  SampleTime=Tmega
  Реж. упр. Местное : Outport  Port=2  SampleTime=Tmega
  wires:
  Logical Operator32/1 -> Logical Operator37/2
  Logical Operator38/1 -> Logical Operator36/2, Logical Operator37/1
  Logical Operator27/1 -> Logical Operator36/1, Logical Operator32/1
  Constant2/1 -> Logical Operator27/2
  Вывод ОУ/1 -> Logical Operator38/1
  Дист. упр./1 -> Logical Operator27/1
  Logical Operator36/1 -> Реж. упр. АСУ/1
  Logical Operator37/1 -> Реж. упр. Местное/1
